simulink model "virtual_aero2_gain_scheduling"  (R2021a)
settings: Solver=ode1  StartTime=0.0  StopTime=inf  FixedStep=0.002  RelTol=1e-3
undefined symbols (not defined in the file): HIL, qc_get_step_size
libraries: quarc_library x10, simulink_extras x2
settings Model: Creator=MLevis  LastModifiedBy=MLevis
settings DataIOCC: ReturnWorkspaceOutputs=off

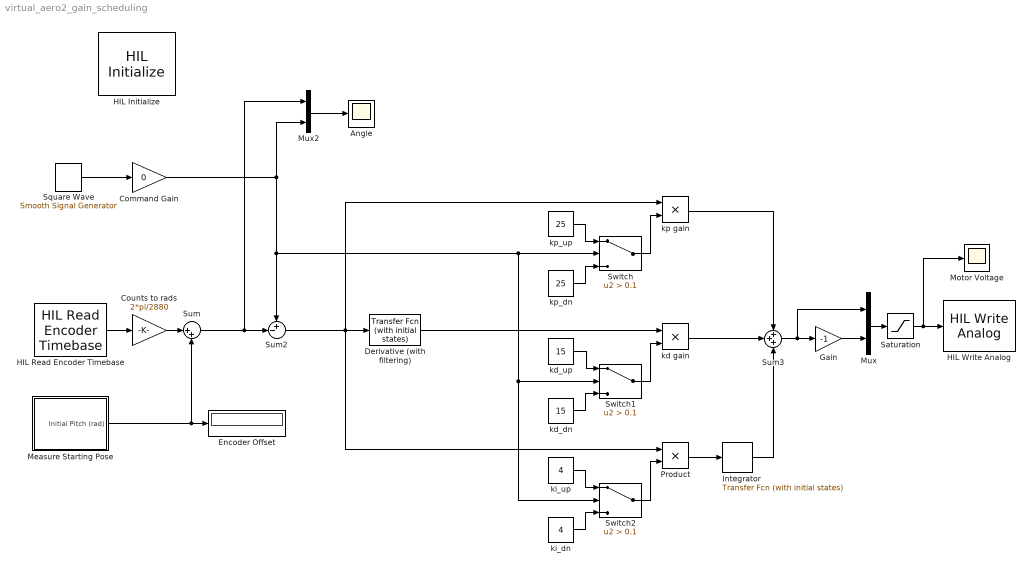
== system virtual_aero2_gain_scheduling ==
  Angle : Scope
  Command Gain : Gain  Gain=0
  Counts to rads : Gain  Gain=2*pi/2880
  Derivative (with filtering) : simulink_extras/Additional Linear/Transfer Fcn (with initial states)  N=[20 0]  D=[1 20]  X0=0
  Encoder Offset : Display
  Gain : Gain  Gain=-1
  HIL Initialize : quarc_library/Data Acquisition/Generic/Configuration/HIL Initialize  Priority=-99  object_name=HIL-1  board_type=quanser_aero2_usb  board_number=0@tcpip://localhost:18950  board_options=""  exclusive=off  active=on  hardware_clocks=[0]  clock_modes=[]  initial_clock_frequencies=[]  set_clock_params_at_start=off  set_clock_params_at_switch_in=off  set_clock_frequencies_at_start=off  set_clock_frequencies_at_switch_in=off  analog_input_channels=[0:1]  analog_input_configurations=[]  analog_input_maximums=3  analog_input_minimums=-3  set_analog_input_params_at_start=off  set_analog_input_params_at_switch_in=off  analog_output_channels=[0:1]  analog_output_maximums=24  analog_output_minimums=-24  initial_analog_outputs=[0]  final_analog_outputs=[0]  watchdog_analog_outputs=[0]  set_analog_output_params_at_start=off  set_analog_output_params_at_switch_in=off  set_analog_outputs_at_start=on  set_analog_outputs_at_switch_in=off  set_analog_outputs_at_terminate=on  set_analog_outputs_at_switch_out=off  set_analog_outputs_on_watchdog=on  digital_input_channels=[]  digital_output_channels=[0:1]  digital_output_configuration=[]  initial_digital_outputs=[1]  final_digital_outputs=[0]  watchdog_digital_outputs=[0]  set_digital_output_params_at_start=off  set_digital_output_params_at_switch_in=off  set_digital_outputs_at_start=on  set_digital_outputs_at_switch_in=off  set_digital_outputs_at_terminate=on  set_digital_outputs_at_switch_out=off  set_digital_outputs_on_watchdog=on  encoder_channels=[0:3]  quadrature=[4]  encoder_filter_frequency=[]  initial_encoder_counts=[0]  set_encoder_params_at_start=off  set_encoder_params_at_switch_in=off  set_encoder_counts_at_start=on  set_encoder_counts_at_switch_in=off  pwm_channels=[]  pwm_modes=[]  pwm_frequency=[]  pwm_configuration=[]  pwm_alignment=[]  pwm_polarity=[]  pwm_leading_deadband=[]  pwm_trailing_deadband=[]  initial_pwm_outputs=[]  final_pwm_outputs=[]  watchdog_pwm_outputs=[]  set_pwm_params_at_start=off  set_pwm_params_at_switch_in=off  set_pwm_outputs_at_start=off  set_pwm_outputs_at_switch_in=off  set_pwm_outputs_at_terminate=off  set_pwm_outputs_at_switch_out=off  set_pwm_outputs_on_watchdog=off  other_output_channels=[11000:11002]  initial_other_outputs=[0 1 0]  final_other_outputs=[1 0 0]  watchdog_other_outputs=[0 0 1]  set_other_outputs_at_start=on  set_other_outputs_at_switch_in=off  set_other_outputs_at_terminate=on  set_other_outputs_at_switch_out=off  set_other_outputs_on_watchdog=on
  HIL Read Encoder Timebase : quarc_library/Data Acquisition/Generic/Timebases/HIL Read Encoder Timebase  object_name=HIL-1  clock=0  channels=2  active=on  vector_output=off  data_type_mode=Inherit via back propagation  data_type=double  overflow_mode=Synchronize (for simulated cards only)  samples_in_buffer=max(ceil(1/qc_get_step_size), 1)
  HIL Write Analog : quarc_library/Data Acquisition/Generic/Immediate I//O/HIL Write Analog  object_name=HIL-1  channels=[0:1]  sample_time=-1  active=on  vector_input=on
  Integrator : simulink_extras/Additional Linear/Transfer Fcn (with initial states)  N=[1]  D=[1 0]  X0=0
  Measure Starting Pose : Subsystem
  Motor Voltage : Scope
  Mux : Mux  Inputs=2
  Mux2 : Mux  Inputs=2
  Product : Product
  Saturation : Saturate  UpperLimit=24  LowerLimit=-24
  Square Wave : quarc_library/Sources/Signals/Smooth Signal Generator  signal_type=Square  source=Internal (dialog parameters)  amplitude=1  frequency=0.05  initial_phase=0  sample_time=qc_get_step_size  output_cos=off
      settings: SourceProductName=QUARC Targets
  Sum : Sum  Inputs=|++
  Sum2 : Sum  Inputs=+-|
  Sum3 : Sum  Inputs=+++
  Switch : Switch  Criteria=u2 > Threshold  Threshold=0.1
  Switch1 : Switch  Criteria=u2 > Threshold  Threshold=0.1
  Switch2 : Switch  Criteria=u2 > Threshold  Threshold=0.1
  kd gain : Product
  kd_dn : Constant  Value=15
  kd_up : Constant  Value=15
  ki_dn : Constant  Value=4
  ki_up : Constant  Value=4
  kp gain : Product
  kp_dn : Constant  Value=25
  kp_up : Constant  Value=25
  wires:
  Product/1 -> Integrator/1
  Integrator/1 -> Sum3/3
  kp gain/1 -> Sum3/1
  HIL Read Encoder Timebase/1 -> Counts to rads/1
  Derivative (with filtering)/1 -> kd gain/1
  Sum2/1 -> Product/1, kp gain/1, Derivative (with filtering)/1
  Command Gain/1 -> Sum2/1, Switch2/2, Switch1/2, Switch/2, Mux2/2
  Sum3/1 -> Mux/1, Gain/1
  Switch1/1 -> kd gain/2
  Sum/1 -> Mux2/1, Sum2/2
  ki_dn/1 -> Switch2/3
  Mux/1 -> Saturation/1
  Measure Starting Pose/1(Initial Pitch (rad)) -> Encoder Offset/1, Sum/2
  kp_dn/1 -> Switch/3
  Counts to rads/1 -> Sum/1
  Mux2/1 -> Angle/1
  Saturation/1 -> Motor Voltage/1, HIL Write Analog/1
  kd_up/1 -> Switch1/1
  kd_dn/1 -> Switch1/3
  Switch2/1 -> Product/2
  kp_up/1 -> Switch/1
  Switch/1 -> kp gain/2
  ki_up/1 -> Switch2/1
  Gain/1 -> Mux/2
  kd gain/1 -> Sum3/2
  Square Wave/1 -> Command Gain/1

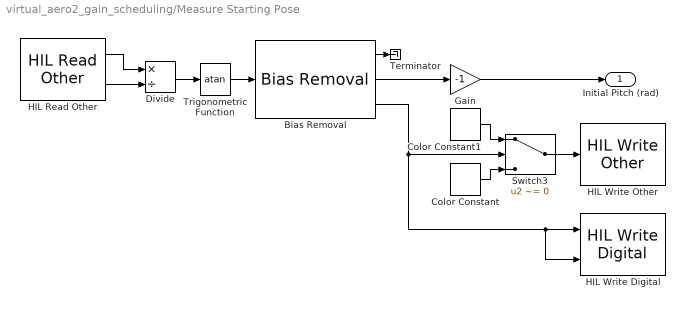
== system virtual_aero2_gain_scheduling/Measure Starting Pose ==
  Bias Removal : quarc_library/Discrete/Bias Removal  start_time=0  end_time=2  switch_id=0  sample_time=qc_get_step_size
      settings: SourceProductName=QUARC Targets
  Color Constant : quarc_library/Sources/Signals/Color Constant  color=[1 1 0]
      settings: SourceProductName=QUARC Targets
  Color Constant1 : quarc_library/Sources/Signals/Color Constant  color=[0 1 0]
      settings: SourceProductName=QUARC Targets
  Divide : Product  Inputs=*/
  Gain : Gain  Gain=-1
  HIL Read Other : quarc_library/Data Acquisition/Generic/Immediate I//O/HIL Read Other  object_name=HIL-1  channels=[4000 4002]  sample_time=qc_get_step_size  active=on  vector_output=off
      settings: AttributesFormatString=(%<object_name>)  SourceProductName=QUARC Targets
  HIL Write Digital : quarc_library/Data Acquisition/Generic/Immediate I//O/HIL Write Digital  object_name=HIL-1  channels=[0:1]  sample_time=-1  active=off  vector_input=off
      settings: SourceProductName=QUARC Targets
  HIL Write Other : quarc_library/Data Acquisition/Generic/Immediate I//O/HIL Write Other  object_name=HIL-1  channels=[11000:11002]  sample_time=-1  active=off  vector_input=on
      settings: AttributesFormatString=(%<object_name>)  SourceProductName=QUARC Targets
  Switch3 : Switch  Criteria=u2 ~= 0
  Terminator : Terminator
  Trigonometric Function : Trigonometry  Operator=atan
  Initial Pitch (rad) : Outport
  wires:
  Color Constant/1 -> Switch3/3
  Bias Removal/1 -> Terminator/1
  Divide/1 -> Trigonometric Function/1
  Trigonometric Function/1 -> Bias Removal/1
  HIL Read Other/2 -> Divide/2
  Bias Removal/3 -> HIL Write Digital/2, HIL Write Digital/1, Switch3/2
  Bias Removal/2 -> Gain/1
  Switch3/1 -> HIL Write Other/1
  HIL Read Other/1 -> Divide/1
  Color Constant1/1 -> Switch3/1
  Gain/1 -> Initial Pitch (rad)/1
